simulink model "third"  (R2018b)
settings: Solver=VariableStepAuto  StartTime=0.0  StopTime=10.0  MaxStep=0.01  RelTol=1e-3
settings Model: Creator=kekos  LastModifiedBy=kekos

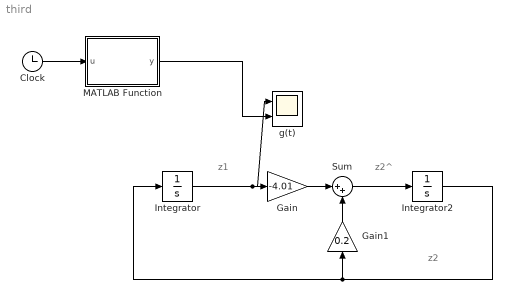
== system third ==
  note: z2
  note: z2^
  note: z1
  Clock : Clock
  Gain : Gain  Gain=-4.01
  Gain1 : Gain  Gain=0.2
  Integrator : Integrator  InitialCondition=1.68
  Integrator2 : Integrator  InitialCondition=2.33
  MATLAB Function : MATLAB Function  TreatAsAtomicUnit=on
  Sum : Sum  Inputs=|++
  g(t) : Scope  NumInputPorts=2
  wires:
  Integrator/1 -> g(t)/1, Gain/1
  Sum/1 -> Integrator2/1
  Integrator2/1 -> Integrator/1, Gain1/1
  Gain/1 -> Sum/1
  Gain1/1 -> Sum/2
  Clock/1 -> MATLAB Function/1(u)
  MATLAB Function/1(y) -> g(t)/2

== matlab function third/MATLAB Function ==
  data: u input; y output
function y = fcn(u)

y = 2*exp(0.1*u)*sin(2*u+1);
